simulink subsystem "DC_gearmotor_resonant_load"  (R2024b)
settings: Solver=VariableStepAuto  StartTime=0.0  StopTime=10.0  RelTol=1e-3
values from neighbouring files (symbols this model uses):
  rads2rpm = 60/2/pi    (= 9.54929658551)    [Plant_ModelParameters.m]
settings Model: Creator=Federico Bergami  LastModifiedBy=Federico Bergami

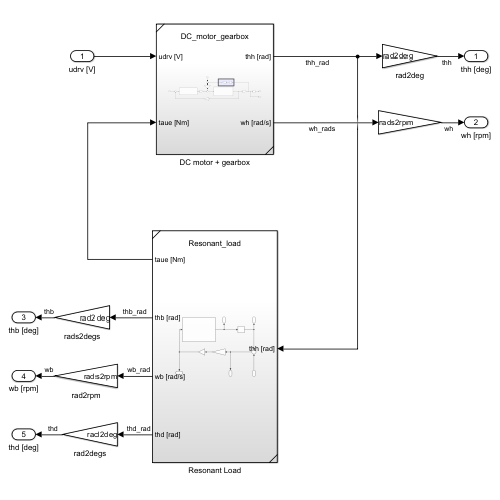
[thumbnail: Simulink's stored preview of the top-level diagram]
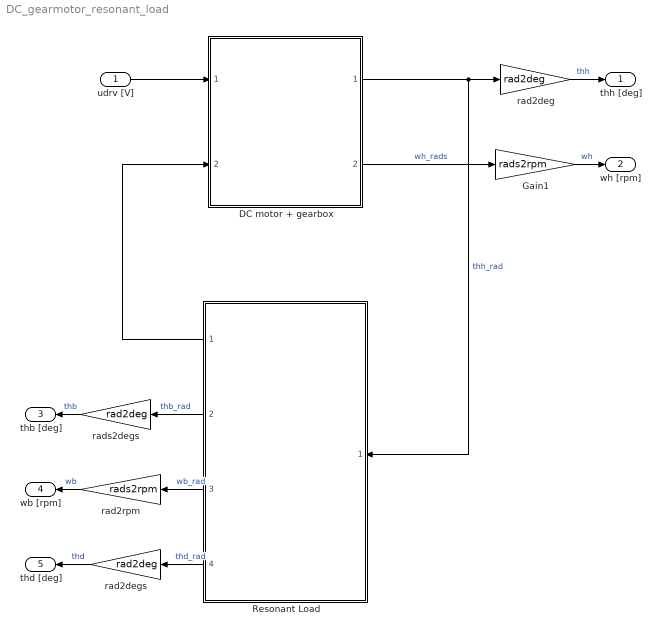
== system DC_gearmotor_resonant_load ==
  udrv [V] : Inport
  DC motor + gearbox : Subsystem  ReferencedSubsystem=DC_motor_gearbox
  Gain1 : Gain  Gain=rads2rpm
  Resonant Load : Subsystem  ReferencedSubsystem=Resonant_load
  rad2deg : Gain  Gain=rad2deg
  rad2degs : Gain  Gain=rad2deg
  rad2rpm : Gain  Gain=rads2rpm
  rads2degs : Gain  Gain=rad2deg
  thh [deg] : Outport
  wh [rpm] : Outport  Port=2
  thb [deg] : Outport  Port=3
  wb [rpm] : Outport  Port=4
  thd [deg] : Outport  Port=5
  wires:
  udrv [V]/1 -> DC motor + gearbox/1
  Resonant Load/1 -> DC motor + gearbox/2
  DC motor + gearbox/1 -> Resonant Load/1, rad2deg/1  "thh_rad"
  rad2deg/1 -> thh [deg]/1  "thh"
  Gain1/1 -> wh [rpm]/1  "wh"
  DC motor + gearbox/2 -> Gain1/1  "wh_rads"
  rads2degs/1 -> thb [deg]/1  "thb"
  rad2rpm/1 -> wb [rpm]/1  "wb"
  rad2degs/1 -> thd [deg]/1  "thd"
  Resonant Load/2 -> rads2degs/1  "thb_rad"
  Resonant Load/3 -> rad2rpm/1  "wb_rad"
  Resonant Load/4 -> rad2degs/1  "thd_rad"
